simulink model "rockets"  (R2013b)
settings: Solver=ode5  StartTime=0.0  StopTime=200  FixedStep=0.001  RelTol=1e-3
libraries: simulink x1
settings Model: Creator=user  LastModifiedBy=user

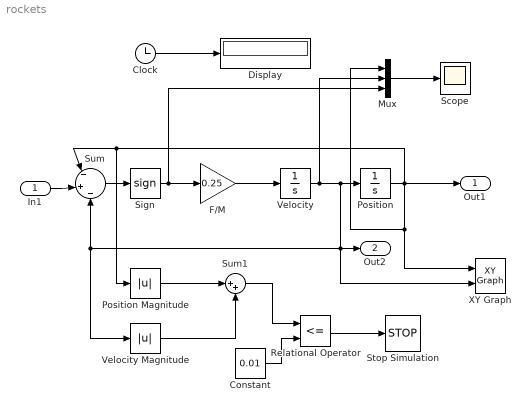
== system rockets ==
  In1 : Inport
  Clock : Clock
  Constant : Constant  Value=0.01
  Display : Display
  F/M : Gain  Gain=0.25
  Mux : Mux  Inputs=3
  Position : Integrator  InitialCondition=-1.5
  Position Magnitude : Abs
  Relational Operator : RelationalOperator  Operator=<=  OutDataTypeStr=boolean
  Scope : Scope
      settings: MaxDataPoints=70000
  Sign : Signum
  Stop Simulation : Stop
  Sum : Sum  Inputs=|-|+|-
  Sum1 : Sum  Inputs=|++
  Velocity : Integrator  InitialCondition=2.5
  Velocity Magnitude : Abs
  XY Graph : simulink/Sinks/XY Graph  xmin=-15  xmax=15  ymin=-5  ymax=5  st=-1
  Out1 : Outport
  Out2 : Outport  Port=2
  wires:
  F/M/1 -> Velocity/1
  Velocity/1 -> Mux/2, XY Graph/2, Out2/1, Sum/3, Velocity Magnitude/1, Position/1
  In1/1 -> Sum/2
  Position/1 -> Mux/1, XY Graph/1, Position Magnitude/1, Sum/1, Out1/1
  Sum/1 -> Sign/1
  Sign/1 -> Mux/3, F/M/1
  Mux/1 -> Scope/1
  Position Magnitude/1 -> Sum1/1
  Velocity Magnitude/1 -> Sum1/2
  Sum1/1 -> Relational Operator/1
  Constant/1 -> Relational Operator/2
  Relational Operator/1 -> Stop Simulation/1
  Clock/1 -> Display/1
